simulink model "Q1_melisa"  (R2016a)
settings: Solver=VariableStepAuto  StartTime=0.0  StopTime=0.05  RelTol=1e-3
libraries: powerlib x36, powerlib_meascontrol x2
settings Model: Creator=syf  LastModifiedBy=syf

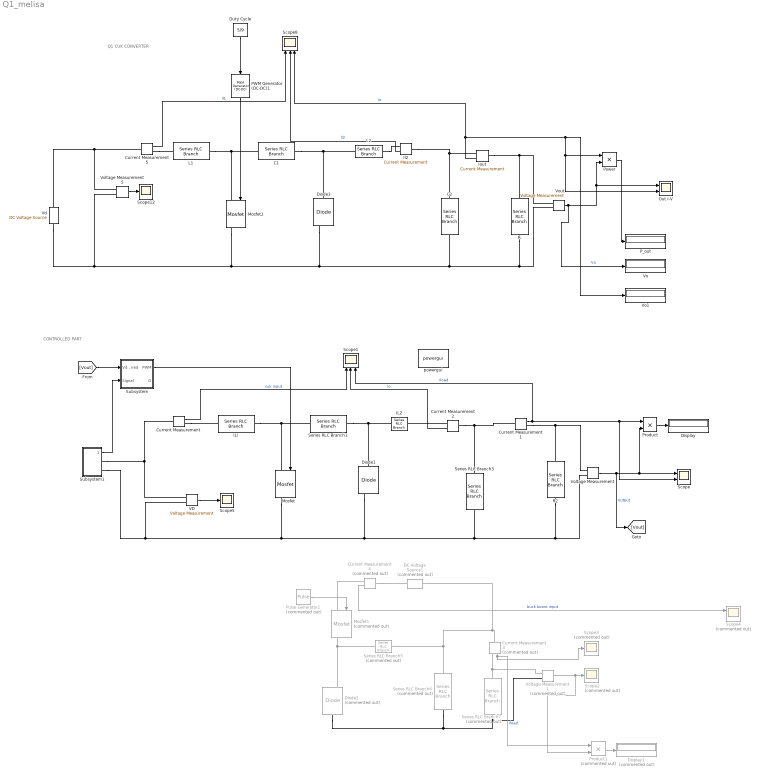
== system Q1_melisa ==
  note: CONTROLLED PART
  note: Q1 CUK CONVERTER
  C1 : powerlib/Elements/Series RLC Branch  LConnTagsString=__new0  RConnTagsString=__new0  BranchType=C  Resistance=1  Inductance=1e-3  SetiL0=off  InitialCurrent=0  Capacitance=9600e-6  Setx0=on  InitialVoltage=25  Measurements=None
  C2 : powerlib/Elements/Series RLC Branch  LConnTagsString=__new0  RConnTagsString=__new0  BranchType=C  Resistance=1  Inductance=1e-3  SetiL0=off  InitialCurrent=0  Capacitance=47e-6  Setx0=on  InitialVoltage=15  Measurements=None
  Current Measurement{,1..2,5} (4 alike) : powerlib/Measurements/Current Measurement  PhasorSimulation=off  OutputType=Complex  PSBequivalent=0
  Current Measurement3 : powerlib/Measurements/Current Measurement  Commented=on  PhasorSimulation=off  OutputType=Complex  PSBequivalent=0
  Current Measurement4 : powerlib/Measurements/Current Measurement  Commented=on  PhasorSimulation=off  OutputType=Complex  PSBequivalent=0
  DC Voltage Source1 : powerlib/Electrical Sources/DC Voltage Source  Commented=on  Amplitude=12  Measurements=None
  Diode1 : powerlib/Power Electronics/Diode  Ron=0.001  Lon=0  Vf=0  IC=0  UseSnubber=off  Rs=500  Cs=250e-9  Measurements=on
  Diode2 : powerlib/Power Electronics/Diode  Commented=on  Ron=0.001  Lon=0  Vf=0  IC=0  UseSnubber=off  Rs=500  Cs=250e-9  Measurements=on
  Diode3 : powerlib/Power Electronics/Diode  Ron=0.001  Lon=0  Vf=0  IC=0  UseSnubber=off  Rs=500  Cs=250e-9  Measurements=on
  Display : Display
  Display1 : Display  Commented=on
  Duty Cycle : Constant  Value=5/9
  IL! : powerlib/Elements/Series RLC Branch  LConnTagsString=__new0  RConnTagsString=__new0  BranchType=L  Resistance=1  Inductance=4.7e-6  SetiL0=off  InitialCurrent=0  Capacitance=1e-6  Setx0=off  InitialVoltage=0  Measurements=None
  IL2 : powerlib/Elements/Series RLC Branch  LConnTagsString=__new0  RConnTagsString=__new0  BranchType=L  Resistance=1  Inductance=5.6e-6  SetiL0=off  InitialCurrent=0  Capacitance=1e-6  Setx0=off  InitialVoltage=0  Measurements=None
  Il2 : powerlib/Measurements/Current Measurement  PhasorSimulation=off  OutputType=Complex  PSBequivalent=0
  Iout : powerlib/Measurements/Current Measurement  PhasorSimulation=off  OutputType=Complex  PSBequivalent=0
  L1 : powerlib/Elements/Series RLC Branch  LConnTagsString=__new0  RConnTagsString=__new0  BranchType=L  Resistance=1  Inductance=4.7e-6  SetiL0=on  InitialCurrent=5  Capacitance=1e-6  Setx0=off  InitialVoltage=0  Measurements=None
  L2 : powerlib/Elements/Series RLC Branch  LConnTagsString=__new0  RConnTagsString=__new0  BranchType=L  Resistance=1  Inductance=5.6e-6  SetiL0=on  InitialCurrent=4  Capacitance=1e-6  Setx0=off  InitialVoltage=0  Measurements=None
  Mosfet : powerlib/Power Electronics/Mosfet  Ron=0.1  Lon=0  Rd=0.01  Vfd=0  IC=0  Rs=1e5  Cs=inf  Measurements=on
  Mosfet1 : powerlib/Power Electronics/Mosfet  Commented=on  Ron=0.1  Lon=0  Rd=0.01  Vfd=0  IC=0  Rs=1e5  Cs=inf  Measurements=on
  Mosfet2 : powerlib/Power Electronics/Mosfet  Ron=0.1  Lon=0  Rd=0.01  Vfd=0  IC=0  Rs=1e5  Cs=inf  Measurements=on
  Out I-V : Scope  NumInputPorts=2
  PWM Generator (DC-DC)1 : powerlib_meascontrol/Pulse & Signal Generators/PWM Generator (DC-DC)  Fsw=150e3  Ts=0
  P_out : Display
  Power : Product
  Product : Product
  Product1 : Product  Commented=on
  Pulse Generator1 : DiscretePulseGenerator  Commented=on  PulseType=Time based  Period=1/(150e3)  PulseWidth=5/9*100
  R : powerlib/Elements/Series RLC Branch  LConnTagsString=__new0  RConnTagsString=__new0  BranchType=R  Resistance=3.75  Inductance=1e-3  SetiL0=off  InitialCurrent=0  Capacitance=1e-6  Setx0=off  InitialVoltage=0  Measurements=None
  R2 : powerlib/Elements/Series RLC Branch  LConnTagsString=__new0  RConnTagsString=__new0  BranchType=R  Resistance=3  Inductance=1e-3  SetiL0=off  InitialCurrent=0  Capacitance=1e-6  Setx0=off  InitialVoltage=0  Measurements=None
  Scope : Scope  NumInputPorts=2
  Scope1 : Scope  NumInputPorts=3
  Scope12 : Scope
  Scope2 : Scope  Commented=on
  Scope3 : Scope  Commented=on
  Scope4 : Scope  Commented=on  NumInputPorts=2
  Scope5 : Scope
  Scope8 : Scope  NumInputPorts=3
  Series RLC Branch1 : powerlib/Elements/Series RLC Branch  LConnTagsString=__new0  RConnTagsString=__new0  BranchType=C  Resistance=1  Inductance=1e-3  SetiL0=off  InitialCurrent=0  Capacitance=9600e-6  Setx0=off  InitialVoltage=0  Measurements=None
  Series RLC Branch3 : powerlib/Elements/Series RLC Branch  LConnTagsString=__new0  RConnTagsString=__new0  BranchType=C  Resistance=1  Inductance=1e-3  SetiL0=off  InitialCurrent=0  Capacitance=47e-6  Setx0=off  InitialVoltage=0  Measurements=None
  Series RLC Branch5 : powerlib/Elements/Series RLC Branch  Commented=on  LConnTagsString=__new0  RConnTagsString=__new0  BranchType=L  Resistance=1  Inductance=22e-6  SetiL0=off  InitialCurrent=0  Capacitance=1e-6  Setx0=off  InitialVoltage=0  Measurements=None
  Series RLC Branch6 : powerlib/Elements/Series RLC Branch  Commented=on  LConnTagsString=__new0  RConnTagsString=__new0  BranchType=C  Resistance=1  Inductance=1e-3  SetiL0=off  InitialCurrent=0  Capacitance=63e-6  Setx0=off  InitialVoltage=0  Measurements=None
  Series RLC Branch7 : powerlib/Elements/Series RLC Branch  Commented=on  LConnTagsString=__new0  RConnTagsString=__new0  BranchType=R  Resistance=3  Inductance=1e-3  SetiL0=off  InitialCurrent=0  Capacitance=1e-6  Setx0=off  InitialVoltage=0  Measurements=None
  Subsystem : Subsystem
  Subsystem1 : Subsystem
  VD : powerlib/Measurements/Voltage Measurement  PhasorSimulation=off  OutputType=Complex  PSBequivalent=0
  Vd : powerlib/Electrical Sources/DC Voltage Source  Amplitude=12  Measurements=None
  Vo : Display
  Vo1 : Display
  Voltage Measurement : powerlib/Measurements/Voltage Measurement  PhasorSimulation=off  OutputType=Complex  PSBequivalent=0
  Voltage Measurement1 : powerlib/Measurements/Voltage Measurement  Commented=on  PhasorSimulation=off  OutputType=Complex  PSBequivalent=0
  Voltage Measurement5 : powerlib/Measurements/Voltage Measurement  PhasorSimulation=off  OutputType=Complex  PSBequivalent=0
  Vout : powerlib/Measurements/Voltage Measurement  PhasorSimulation=off  OutputType=Complex  PSBequivalent=0
  powergui : powerlib/powergui  Priority=1  SimulationMode=Continuous  SolverType=Tustin/Backward Euler (TBE)  SampleTime=50e-6  frequency=60  SPID=on  DisableSnubberDevices=off  DisableRonSwitches=off  DisableVfSwitches=off  SwTol=0  DisplayEquations=off  Interpol=off  ExternalGateDelay=off  methode=off  Ts=10  FunctionMessages=off  echomessages=off  HookPort=off  EnableUseOfTLC=off  x0status=blocks  frequencyindice=0  Pbase=100e6  ErrMax=1e-4  Iterations=50  UnitsV=kV  UnitsW=MW  buscounter=0  RestoreLinks=warning  ResistiveCurrentMeasurement=off  Frange=[0:2:500]  Ylog=off  Xlog=on  ShowGrid=off  save=off  variable=ZData  structure=0  ZoomFFT=off  StartTime=0.0  cycles=1  DisplayStyle=1  fundamental=60  FreqAxis=off  MaxFrequency=1000  frequencyindicesteady=1  RmsSteady=1  display=off
  wires:
  Current Measurement1/1 -> Scope/2, Product/1, Scope1/3  "Iload"
  Current Measurement/1 -> Scope1/1  "cuk input"
  Product/1 -> Display/1
  Current Measurement2/1 -> Scope1/2  "Io"
  Pulse Generator1/1 -> Mosfet1/1
  Voltage Measurement1/1 -> Product1/2, Scope2/1
  Current Measurement3/1 -> Product1/1, Scope3/1  "Iload"
  Product1/1 -> Display1/1
  Current Measurement4/1 -> Scope4/1  "buck boost input"
  VD/1 -> Scope5/1
  Voltage Measurement/1 -> [Vout], Product/2, Scope/1  "output"
  PWM Generator (DC-DC)1/1 -> Mosfet2/1
  Iout/1 -> Vo1/1, Out I-V/2, Power/1, Scope8/3  "Io"
  Current Measurement5/1 -> Scope8/1  "Il1"
  Power/1 -> P_out/1
  Il2/1 -> Scope8/2  "Il2"
  Voltage Measurement5/1 -> Scope12/1
  Vout/1 -> Vo/1, Power/2, Out I-V/1  "Vo"
  Duty Cycle/1 -> PWM Generator (DC-DC)1/1
  [Vout] -> Subsystem/1(Vdesired)
  Subsystem/1(PWM) -> Mosfet/1
  Subsystem1/1(Signal) -> Subsystem/2(Signal)
  connections:
  Current Measurement1/LConn1 -- Current Measurement2/LConn1 -- Series RLC Branch3/LConn1
  Series RLC Branch1/RConn1 -- IL2/RConn1 -- Diode1/LConn1
  IL!/RConn1 -- Series RLC Branch1/LConn1 -- Mosfet/LConn1
  Mosfet/RConn1 -- Diode1/RConn1 -- R2/LConn1 -- Voltage Measurement/LConn2 -- Series RLC Branch3/RConn1 -- Subsystem1/RConn2 -- VD/LConn2
  Current Measurement/RConn1 -- IL!/LConn1
  Current Measurement1/RConn1 -- R2/RConn1 -- Voltage Measurement/LConn1
  Current Measurement2/RConn1 -- IL2/LConn1
  Mosfet1/RConn1 -- Diode2/RConn1 -- Series RLC Branch5/LConn1
  Series RLC Branch5/RConn1 -- Series RLC Branch6/LConn1 -- Current Measurement3/LConn1 -- DC Voltage Source1/LConn1
  Diode2/LConn1 -- Series RLC Branch6/RConn1 -- Voltage Measurement1/LConn2 -- Series RLC Branch7/RConn1
  Voltage Measurement1/LConn1 -- Series RLC Branch7/LConn1 -- Current Measurement3/RConn1
  Current Measurement4/LConn1 -- DC Voltage Source1/RConn1
  Current Measurement4/RConn1 -- Mosfet1/LConn1
  Iout/RConn1 -- Il2/LConn1 -- C2/LConn1
  Diode3/LConn1 -- C1/RConn1 -- L2/RConn1
  L1/RConn1 -- C1/LConn1 -- Mosfet2/LConn1
  Voltage Measurement5/LConn2 -- Vout/LConn1 -- R/LConn1 -- C2/RConn1 -- Diode3/RConn1 -- Mosfet2/RConn1 -- Vd/LConn1
  Voltage Measurement5/LConn1 -- Current Measurement5/LConn1 -- Vd/RConn1
  Iout/LConn1 -- Vout/LConn2 -- R/RConn1
  Current Measurement5/RConn1 -- L1/LConn1
  L2/LConn1 -- Il2/RConn1
  VD/LConn1 -- Subsystem1/RConn1 -- Current Measurement/LConn1

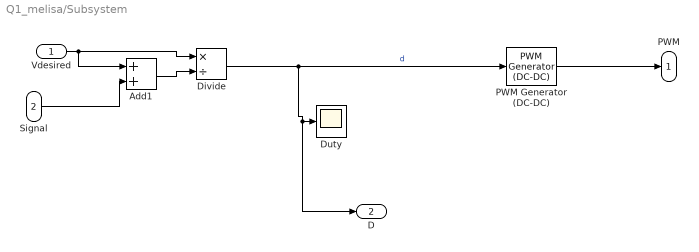
== system Q1_melisa/Subsystem ==
  Vdesired : Inport
  Signal : Inport  Port=2
  Add1 : Sum
  Divide : Product  Inputs=*/
  Duty : Scope
  PWM Generator (DC-DC) : powerlib_meascontrol/Pulse & Signal Generators/PWM Generator (DC-DC)  Fsw=150e3  Ts=0
  PWM : Outport
  D : Outport  Port=2
  wires:
  PWM Generator (DC-DC)/1 -> PWM/1
  Signal/1 -> Add1/2
  Divide/1 -> D/1, Duty/1, PWM Generator (DC-DC)/1  "d"
  Add1/1 -> Divide/2
  Vdesired/1 -> Add1/1, Divide/1

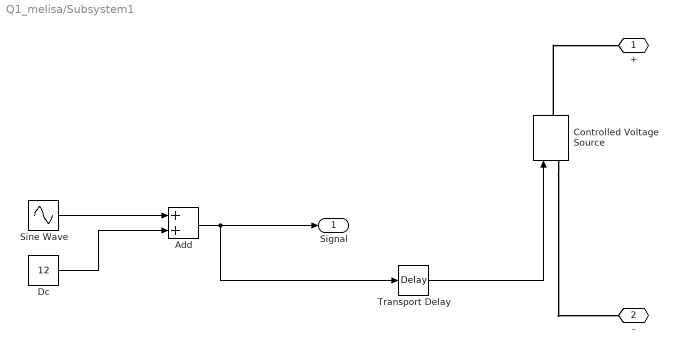
== system Q1_melisa/Subsystem1 ==
  Add : Sum
  Controlled Voltage Source : powerlib/Electrical Sources/Controlled Voltage Source  Initialize=on  Source_Type=DC  Amplitude=0  Phase=0  Frequency=300  Measurements=None
  Dc : Constant  Value=12
  Sine Wave : Sin  Amplitude=2  Frequency=600*pi  SampleTime=0
  Transport Delay : TransportDelay  DelayTime=2e-4
  + : PMIOPort  Port=1  Side=Right
  - : PMIOPort  Port=2  Side=Right
  Signal : Outport
  wires:
  Transport Delay/1 -> Controlled Voltage Source/1
  Dc/1 -> Add/2
  Sine Wave/1 -> Add/1
  Add/1 -> Transport Delay/1, Signal/1
  connections:
  Controlled Voltage Source/RConn1 -- +/RConn1
  Controlled Voltage Source/LConn1 -- -/RConn1
